simulink model "Assign_Task1and2"  (R2024a)
settings: Solver=ode1  StartTime=0.0  StopTime=simTime  FixedStep=Ts  MaxStep=Ts  RelTol=1e-3
model workspace (MAT data in the model file):
  wsw = 2000
values from neighbouring files (symbols this model uses):
  fg = 50    [Parameters.m]
  S0non = 1000e6    (= 1000000000)    [Parameters.m]
  simTime = 60    [Parameters.m]
  Ts = 20e-6    (= 2e-05)    [Parameters.m]
  Vhv = 22e3    (= 22000)    [Parameters.m]
  Vmv = 22e3    (= 22000)    [Parameters.m]
libraries: simulink_extras x8, spsCurrentMeasurementLib x6, spsGroundLib x6, spsVoltageMeasurementLib x6, spsThreePhaseParallelRLCLoadLib x5, spsPower3phInstantaneousLib x2, spsSynchronousMachinepuStandardLib x2, spsThreePhaseBreakerLib x1, spsThreePhaseSourceLib x1, sps_lib x1
settings Model: Creator=Vinicius  LastModifiedBy=citcea
settings SolverCC: AlgebraicLoopSolver=TrustRegion
settings DataIOCC: InitialState=out_EMTsteady50VSC.xFinal  SaveOperatingPoint=on  SaveOutput=off  SignalLogging=off  DSMLogging=off  TimeSaveName=t
settings OptimizationCC: BlockReduction=off
settings ModelReferenceCC: EnableRefExpFcnMdlSchedulingChecks=on
settings RTWCC: BuildConfiguration=Faster Runs  GPUComputeCapability=3.5  DLArmComputeVersion=19.05

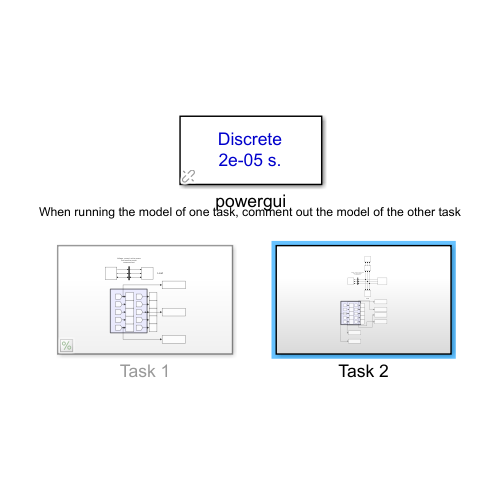
[thumbnail: Simulink's stored preview of the top-level diagram]
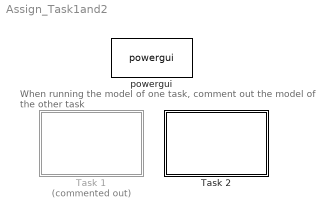
== system Assign_Task1and2 ==
  note: When running the model of one task, comment out the model of the other task
  Task 1 : Subsystem  Commented=on
  Task 2 : Subsystem
  powergui : sps_lib/powergui  Priority=1  SimulationMode=Discrete  SampleTime=Ts  frequency=60  Iterations=50  frequencyindice=50  Pbase=100e6  ErrMax=0.0001  UnitsV=kV  UnitsW=MW  buscounter=0  FunctionMessages=off  echomessages=off  EnableUseOfTLC=off  CurrentSourceSwitches=off  DisableSnubberDevices=off  DisableRonSwitches=off  DisableVfSwitches=off  DisplayEquations=off  AutomaticDiscreteSolvers=off  SolverType=Tustin/Backward Euler (TBE)  Interpol=off  ExternalGateDelay=off  methode=off  Ts=100  x0status=blocks  SPID=on  SwTol=0  HookPort=off  NonlinearTolerance=1e-4  nMaxIteration=100  ContinueOnMaxIteration=off  RestoreLinks=warning  ResistiveCurrentMeasurement=off  Frange=[0:2:500]  Ylog=off  Xlog=on  ShowGrid=off  save=off  variable=ZData  structure=0  ZoomFFT=off  StartTime=0.0  cycles=1  DisplayStyle=1  fundamental=60  FreqAxis=off  MaxFrequency=1000  frequencyindicesteady=1  RmsSteady=1  display=off

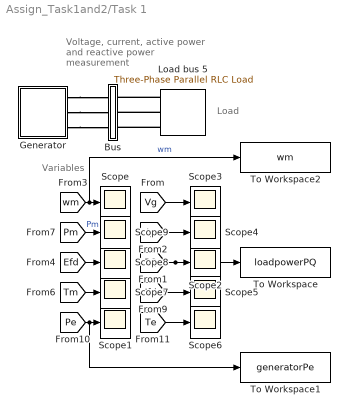
== system Assign_Task1and2/Task 1 ==
  note: Variables
  note: Voltage, current, active power and reactive power measurement
  note: Load
  Bus : Subsystem
  Generator : Subsystem
      mask Display: disp('SG')
  Load bus 5 : spsThreePhaseParallelRLCLoadLib/Three-Phase Parallel RLC Load  LConnTagsString=A|B|C  Configuration=Y (grounded)  NominalVoltage=Vmv  Vabc=[1e3 1e3 1e3]  Vabcp=[1e3 1e3 1e3]  NominalFrequency=fg  UnbalancedPower=off  ActivePower=load_active_power  InductivePower=load_inductive_power  CapacitivePower=load_capacitive_power  Pabc=[10e3 9e3 11e3]  QLabc=[100 90 110]  QCabc=[100 90 110]  Pabcp=[10e3 9e3 11e3]  QLabcp=[100 90 110]  QCabcp=[100 90 110]  Measurements=None  LoadType=constant PQ
  Scope{,1..9} (10 alike) : Scope
  To Workspace : ToWorkspace  VariableName=loadpowerPQ  SaveFormat=Timeseries  SampleTime=-1
  To Workspace1 : ToWorkspace  VariableName=generatorPe  SaveFormat=Timeseries  SampleTime=-1
  To Workspace2 : ToWorkspace  VariableName=wm  SaveFormat=Timeseries  SampleTime=-1
  wires:
  [wm] -> To Workspace2/1, Scope/1  "wm"
  [Pe] -> To Workspace1/1, Scope1/1
  [PQ] -> To Workspace/1, Scope2/1
  [Vg] -> Scope3/1
  [Ig] -> Scope4/1
  [Ifd] -> Scope5/1
  [Te] -> Scope6/1
  [Tm] -> Scope7/1
  [Efd] -> Scope8/1
  [Pm] -> Scope9/1  "Pm"
  connections:
  Load bus 5/LConn1 -- Bus/RConn1
  Load bus 5/LConn2 -- Bus/RConn2
  Generator/RConn1 -- Bus/LConn1
  Load bus 5/LConn3 -- Bus/RConn3
  Generator/RConn2 -- Bus/LConn2
  Generator/RConn3 -- Bus/LConn3

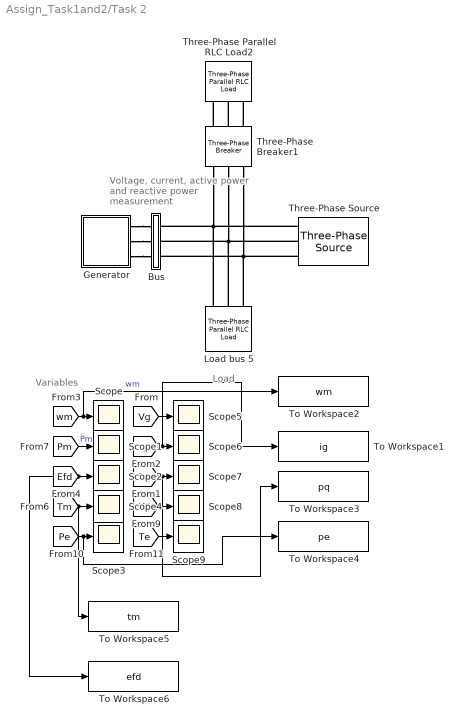
== system Assign_Task1and2/Task 2 ==
  note: Variables
  note: Voltage, current, active power and reactive power measurement
  note: Load
  Bus : Subsystem
  Generator : Subsystem
      mask Display: disp('SG')
  Load bus 5 : spsThreePhaseParallelRLCLoadLib/Three-Phase Parallel RLC Load  LConnTagsString=A|B|C  Configuration=Y (grounded)  NominalVoltage=Vmv  Vabc=[1e3 1e3 1e3]  Vabcp=[1e3 1e3 1e3]  NominalFrequency=fg  UnbalancedPower=off  ActivePower=first_load_active_power  InductivePower=first_load_inductive_power  CapacitivePower=first_load_capacitive_power  Pabc=[10e3 9e3 11e3]  QLabc=[100 90 110]  QCabc=[100 90 110]  Pabcp=[10e3 9e3 11e3]  QLabcp=[100 90 110]  QCabcp=[100 90 110]  Measurements=None  LoadType=constant PQ
  Scope{,1..9} (10 alike) : Scope
  Three-Phase Parallel RLC Load2 : spsThreePhaseParallelRLCLoadLib/Three-Phase Parallel RLC Load  LConnTagsString=A|B|C  Configuration=Y (grounded)  NominalVoltage=Vmv  Vabc=[1 1 1]*Vhv  Vabcp=[1e3 1e3 1e3]  NominalFrequency=fg  UnbalancedPower=off  ActivePower=external_load_active_power  InductivePower=external_load_inductive_power  CapacitivePower=external_load_capacitive_power  Pabc=[10 10 10]*1e6  QLabc=[1 1 1]*1e6  QCabc=[0 0 0]  Pabcp=[10e3 9e3 11e3]  QLabcp=[100 90 110]  QCabcp=[100 90 110]  Measurements=None  LoadType=constant Z
  Three-Phase Breaker1 : spsThreePhaseBreakerLib/Three-Phase Breaker  InitialState=open  SwitchA=on  SwitchB=on  SwitchC=on  SwitchTimes=simTime/2  External=off  BreakerResistance=0.001  SnubberResistance=1e7  SnubberCapacitance=inf  Measurements=None
  Three-Phase Source : spsThreePhaseSourceLib/Three-Phase Source  InternalConnection=Yg  VoltagePhases=off  Voltage=Vmv  PhaseAngle=0  Voltage_phases=[25e3 25e3 25e3]/sqrt(3)  PhaseAngles_phases=[0 -120 +120]  Frequency=50  NonIdealSource=on  SpecifyImpedance=on  Resistance=0.8929  Inductance=16.58e-3  ShortCircuitLevel=Shortcircuit_power  BaseVoltage=Vmv  XRratio=10  BusType=swing  Pref=10e3  Qref=0  Prefabc=[10e3, 10e3, 10e3]  Qrefabc=[0, 0, 0]  Qmin=-inf  Qmax=inf
  To Workspace1 : ToWorkspace  VariableName=ig  SaveFormat=Timeseries  SampleTime=-1
  To Workspace2 : ToWorkspace  VariableName=wm  SaveFormat=Timeseries  SampleTime=-1
  To Workspace3 : ToWorkspace  VariableName=pq  SaveFormat=Timeseries  SampleTime=-1
  To Workspace4 : ToWorkspace  VariableName=pe  SaveFormat=Timeseries  SampleTime=-1
  To Workspace5 : ToWorkspace  VariableName=tm  SaveFormat=Timeseries  SampleTime=-1
  To Workspace6 : ToWorkspace  VariableName=efd  SaveFormat=Timeseries  SampleTime=-1
  wires:
  [wm] -> To Workspace2/1, Scope/1  "wm"
  [Pm] -> Scope1/1  "Pm"
  [Efd] -> To Workspace6/1, Scope2/1
  [Tm] -> To Workspace5/1, Scope4/1
  [Pe] -> To Workspace4/1, Scope3/1
  [Vg] -> Scope5/1
  [Ig] -> To Workspace1/1, Scope6/1
  [PQ] -> To Workspace3/1, Scope7/1
  [Ifd] -> Scope8/1
  [Te] -> Scope9/1
  connections:
  Load bus 5/LConn1 -- Three-Phase Source/RConn1 -- Three-Phase Breaker1/LConn1 -- Bus/RConn1
  Load bus 5/LConn2 -- Three-Phase Source/RConn2 -- Three-Phase Breaker1/LConn2 -- Bus/RConn2
  Generator/RConn1 -- Bus/LConn1
  Load bus 5/LConn3 -- Three-Phase Source/RConn3 -- Three-Phase Breaker1/LConn3 -- Bus/RConn3
  Generator/RConn2 -- Bus/LConn2
  Generator/RConn3 -- Bus/LConn3
  Three-Phase Breaker1/RConn1 -- Three-Phase Parallel RLC Load2/LConn1
  Three-Phase Breaker1/RConn2 -- Three-Phase Parallel RLC Load2/LConn2
  Three-Phase Breaker1/RConn3 -- Three-Phase Parallel RLC Load2/LConn3

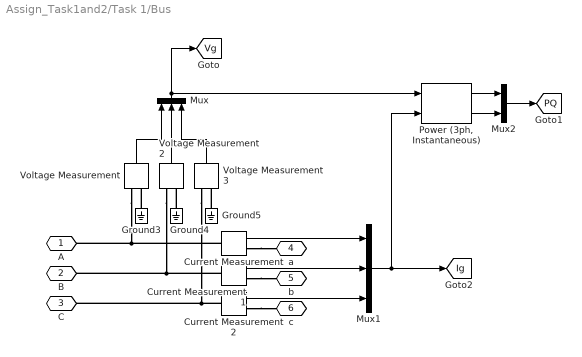
== system Assign_Task1and2/Task 1/Bus ==
  Current Measurement : spsCurrentMeasurementLib/Current Measurement  PhasorSimulation=off  OutputType=Complex  PSBequivalent=0
  Current Measurement1 : spsCurrentMeasurementLib/Current Measurement  PhasorSimulation=off  OutputType=Complex  PSBequivalent=0
  Current Measurement2 : spsCurrentMeasurementLib/Current Measurement  PhasorSimulation=off  OutputType=Complex  PSBequivalent=0
  Ground3 : spsGroundLib/Ground  LConnTagsString=a
  Ground4 : spsGroundLib/Ground  LConnTagsString=a
  Ground5 : spsGroundLib/Ground  LConnTagsString=a
  Mux : Mux  Inputs=3
  Mux1 : Mux  Inputs=3
  Mux2 : Mux  Inputs=2
  "Power (3ph, Instantaneous)" : spsPower3phInstantaneousLib/Power (3ph, Instantaneous)
  Voltage Measurement : spsVoltageMeasurementLib/Voltage Measurement  PhasorSimulation=off  OutputType=Complex  PSBequivalent=0
  Voltage Measurement2 : spsVoltageMeasurementLib/Voltage Measurement  PhasorSimulation=off  OutputType=Complex  PSBequivalent=0
  Voltage Measurement3 : spsVoltageMeasurementLib/Voltage Measurement  PhasorSimulation=off  OutputType=Complex  PSBequivalent=0
  A : PMIOPort  Side=Left
  B : PMIOPort  Port=2  Side=Left
  C : PMIOPort  Port=3  Side=Left
  a : PMIOPort  Port=4  Side=Right
  b : PMIOPort  Port=5  Side=Right
  c : PMIOPort  Port=6  Side=Right
  tag scope: Ig=global, PQ=global, Vg=global
  wires:
  Voltage Measurement3/1 -> Mux/3
  Voltage Measurement2/1 -> Mux/2
  Voltage Measurement/1 -> Mux/1
  Mux/1 -> [Vg], "Power (3ph, Instantaneous)"/1
  Current Measurement/1 -> Mux1/1
  Current Measurement1/1 -> Mux1/2
  Current Measurement2/1 -> Mux1/3
  Mux1/1 -> [Ig], "Power (3ph, Instantaneous)"/2
  "Power (3ph, Instantaneous)"/1 -> Mux2/1
  "Power (3ph, Instantaneous)"/2 -> Mux2/2
  Mux2/1 -> [PQ]
  connections:
  Ground5/LConn1 -- Voltage Measurement3/LConn2
  Current Measurement/RConn1 -- a/RConn1
  Voltage Measurement2/LConn1 -- Current Measurement1/LConn1 -- B/RConn1
  Voltage Measurement3/LConn1 -- Current Measurement2/LConn1 -- C/RConn1
  Voltage Measurement/LConn1 -- Current Measurement/LConn1 -- A/RConn1
  Ground3/LConn1 -- Voltage Measurement/LConn2
  Ground4/LConn1 -- Voltage Measurement2/LConn2
  Current Measurement1/RConn1 -- b/RConn1
  Current Measurement2/RConn1 -- c/RConn1

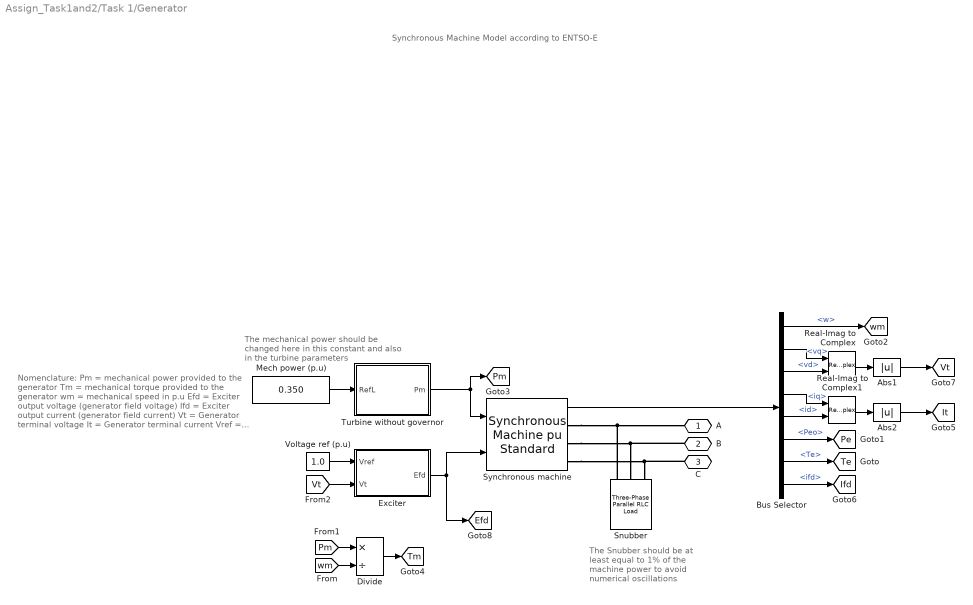
== system Assign_Task1and2/Task 1/Generator ==
  note: The Snubber should be at least equal to 1% of the machine power to avoid numerical oscillations
  note: Nomenclature:
      |
      | Pm = mechanical power provided to the generator
      | Tm = mechanical torque provided to the generator
      | wm = mechanical speed in p.u
      | Efd = Exciter output voltage (generator field voltage)
      | Ifd = Exciter output current (generator field current)
      | Vt = Generator terminal voltage
      | It = Generator terminal current
      | Vref = Voltage regulator reference signal
  note: Synchronous Machine Model according to ENTSO-E
  note: The mechanical power should be changed here in this constant and also in the turbine parameters
  Abs1 : Abs  SaturateOnIntegerOverflow=off
  Abs2 : Abs  SaturateOnIntegerOverflow=off
  Bus Selector : BusSelector  OutputSignals=w,vq,vd,iq,id,Peo,Te,ifd
  Divide : Product  Inputs=*/
  Exciter : Subsystem  mask{K=200, Ta=3, Tb=10, Te=0.05, Emin=-4, Emax=4, Vf0=1.30534}
      mask prompts: K "Controller gain (K)"; Ta "Filter derivative time constant (Ta)(sec)"; Tb "Filter delay time (Tb)(sec)"; Te "Exciter time constant (Te)(sec)"; Emin "Controller minimum output (Emin)"; Emax "Controller maximum output (Emax)"; Vf0 "Initial output (p.u)"
      mask Display:
      | disp('AVR')
      | 
      | port_label('input',1,'Vref')
      | port_label('input',2,'Vc')
      | 
      | port_label('output',1,'Efd')
  Mech power (p.u) : Constant  Value=0.350  VectorParams1D=off
  Real-Imag to Complex : RealImagToComplex
  Real-Imag to Complex1 : RealImagToComplex
  Snubber : spsThreePhaseParallelRLCLoadLib/Three-Phase Parallel RLC Load  LConnTagsString=A|B|C  Configuration=Y (grounded)  NominalVoltage=Vmv  Vabc=[1 1 1]*Vmv  Vabcp=[1e3 1e3 1e3]  NominalFrequency=fg  UnbalancedPower=off  ActivePower=0.05*S0non  InductivePower=0  CapacitivePower=0  Pabc=[10e3 10e3 10e3]  QLabc=[0 0 0]  QCabc=[0 0 0]  Pabcp=[10e3 9e3 11e3]  QLabcp=[100 90 110]  QCabcp=[100 90 110]  Measurements=None  LoadType=constant Z
  Synchronous machine : spsSynchronousMachinepuStandardLib/Synchronous Machine pu Standard  PresetModel=No  MechanicalLoad=Mechanical power Pm  ShowDetailedParameters=on  RotorType=Salient-pole  Units=per unit standard parameters  MeasurementBus=on  NominalParameters=[S0non Vmv fg]  Reactances1=[ 1.81, 0.3, 0.23, 1.76, 0.65, 0.25, 0.15 ]  Reactances2=[2.0 0.35 0.25 1.8 0.3 0.15]  dAxisTimeConstants=Short-circuit  qAxisTimeConstants=Short-circuit  TimeConstants1="[ 4.4849  0.0681  0.1  ]"  TimeConstants2=[ 8.0, 0.03, 1.0, 0.07 ]  TimeConstants3="[  4.49  0.0681  0.0513  ]"  TimeConstants4=[ 8.0, 0.03, 0.3371, 0.0295 ]  TimeConstants5=[ 1.01, 0.053, 0.1 ]  TimeConstants6=[ 1.3201, 0.023, 1.0, 0.07 ]  TimeConstants7=[0.9 0.03 0.05]  TimeConstants8=[ 1.3201, 0.0231, 0.3371, 0.0295 ]  StatorResistance=0.01  Mechanical=[6 0 2]  PolePairs=20  InitialConditions=[0 -60.0721 0.353553 0.353553 0.353553 -8.1301 -128.13 111.87 1.30534]  SetSaturation=off  Saturation=[0.6404,0.7127,0.8441,0.9214,0.9956,1.082,1.19,1.316,1.457;0.7,0.7698,0.8872,0.9466,0.9969,1.046,1.1,1.151,1.201]  LoadFlowParameters=[2 47500000 0 0 0]  TsPowergui=0  TsBlock=-1  IterativeModel=Trapezoidal non iterative  IterativeDiscreteModel=Trapezoidal non iterative  BusType=swing  Pref=475e6  Qref=0  Qmin=-inf  Qmax=inf  PLF=0  QLF=0
  Turbine without governor : Subsystem  mask{R=0.05, T1=0.5, T2=3, T3=10, Dt=0, Vmin=0, Vmax=10, P0=0.350}
      mask prompts: R "Controller droop (R)"; T1 "Governor time constant (T1)(sec)"; T2 "Turbine derivative time constant (T2)(sec)"; T3 "Turbine delay time constant (T3)(sec)"; Dt "Frictional losses factor (Dt)"; Vmin "Minimum gate limit (Vmin)(p.u)"; Vmax "Maximum gate limit (Vmax)(p.u)"; P0 "Initial power (p.u)"
      mask Display:
      | disp('Turbine')
      | 
      | port_label('input',1,'Pref')
      | 
      | port_label('output',1,'Pm')
  Voltage ref (p.u) : Constant  Value=1.0
  A : PMIOPort  Side=Right
  B : PMIOPort  Port=2  Side=Right
  C : PMIOPort  Port=3  Side=Right
  tag scope: Efd=global, Ifd=global, It=global, Pe=global, Pm=global, Te=global, Tm=global, Vt=global, wm=global
  wires:
  Exciter/1(Efd) -> Synchronous machine/2, [Efd]
  Voltage ref (p.u)/1 -> Exciter/1(Vref)
  Turbine without governor/1(Pm) -> Synchronous machine/1, [Pm]
  Mech power (p.u)/1 -> Turbine without governor/1(RefL)
  [Pm] -> Divide/1
  [wm] -> Divide/2
  Divide/1 -> [Tm]
  Bus Selector/3 -> Real-Imag to Complex/2  "<vd>"
  Abs2/1 -> [It]
  Real-Imag to Complex1/1 -> Abs2/1
  Real-Imag to Complex/1 -> Abs1/1
  Bus Selector/5 -> Real-Imag to Complex1/2  "<id>"
  Bus Selector/1 -> [wm]  "<w>"
  Bus Selector/7 -> [Te]  "<Te>"
  Bus Selector/2 -> Real-Imag to Complex/1  "<vq>"
  Bus Selector/6 -> [Pe]  "<Peo>"
  Bus Selector/4 -> Real-Imag to Complex1/1  "<iq>"
  Synchronous machine/1 -> Bus Selector/1
  Bus Selector/8 -> [Ifd]  "<ifd>"
  Abs1/1 -> [Vt]
  [Vt] -> Exciter/2(Vt)
  connections:
  B/RConn1 -- Synchronous machine/RConn2 -- Snubber/LConn2
  C/RConn1 -- Synchronous machine/RConn3 -- Snubber/LConn3
  Snubber/LConn1 -- Synchronous machine/RConn1 -- A/RConn1

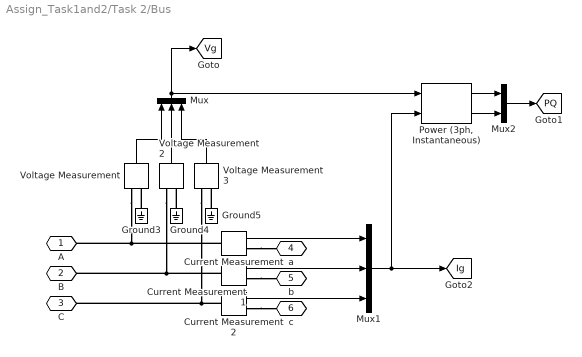
== system Assign_Task1and2/Task 2/Bus ==
  Current Measurement : spsCurrentMeasurementLib/Current Measurement  PhasorSimulation=off  OutputType=Complex  PSBequivalent=0
  Current Measurement1 : spsCurrentMeasurementLib/Current Measurement  PhasorSimulation=off  OutputType=Complex  PSBequivalent=0
  Current Measurement2 : spsCurrentMeasurementLib/Current Measurement  PhasorSimulation=off  OutputType=Complex  PSBequivalent=0
  Ground3 : spsGroundLib/Ground  LConnTagsString=a
  Ground4 : spsGroundLib/Ground  LConnTagsString=a
  Ground5 : spsGroundLib/Ground  LConnTagsString=a
  Mux : Mux  Inputs=3
  Mux1 : Mux  Inputs=3
  Mux2 : Mux  Inputs=2
  "Power (3ph, Instantaneous)" : spsPower3phInstantaneousLib/Power (3ph, Instantaneous)
  Voltage Measurement : spsVoltageMeasurementLib/Voltage Measurement  PhasorSimulation=off  OutputType=Complex  PSBequivalent=0
  Voltage Measurement2 : spsVoltageMeasurementLib/Voltage Measurement  PhasorSimulation=off  OutputType=Complex  PSBequivalent=0
  Voltage Measurement3 : spsVoltageMeasurementLib/Voltage Measurement  PhasorSimulation=off  OutputType=Complex  PSBequivalent=0
  A : PMIOPort  Side=Left
  B : PMIOPort  Port=2  Side=Left
  C : PMIOPort  Port=3  Side=Left
  a : PMIOPort  Port=4  Side=Right
  b : PMIOPort  Port=5  Side=Right
  c : PMIOPort  Port=6  Side=Right
  tag scope: Ig=global, PQ=global, Vg=global
  wires:
  Voltage Measurement3/1 -> Mux/3
  Voltage Measurement2/1 -> Mux/2
  Voltage Measurement/1 -> Mux/1
  Mux/1 -> [Vg], "Power (3ph, Instantaneous)"/1
  Current Measurement/1 -> Mux1/1
  Current Measurement1/1 -> Mux1/2
  Current Measurement2/1 -> Mux1/3
  Mux1/1 -> [Ig], "Power (3ph, Instantaneous)"/2
  "Power (3ph, Instantaneous)"/1 -> Mux2/1
  "Power (3ph, Instantaneous)"/2 -> Mux2/2
  Mux2/1 -> [PQ]
  connections:
  Ground5/LConn1 -- Voltage Measurement3/LConn2
  Current Measurement/RConn1 -- a/RConn1
  Voltage Measurement2/LConn1 -- Current Measurement1/LConn1 -- B/RConn1
  Voltage Measurement3/LConn1 -- Current Measurement2/LConn1 -- C/RConn1
  Voltage Measurement/LConn1 -- Current Measurement/LConn1 -- A/RConn1
  Ground3/LConn1 -- Voltage Measurement/LConn2
  Ground4/LConn1 -- Voltage Measurement2/LConn2
  Current Measurement1/RConn1 -- b/RConn1
  Current Measurement2/RConn1 -- c/RConn1

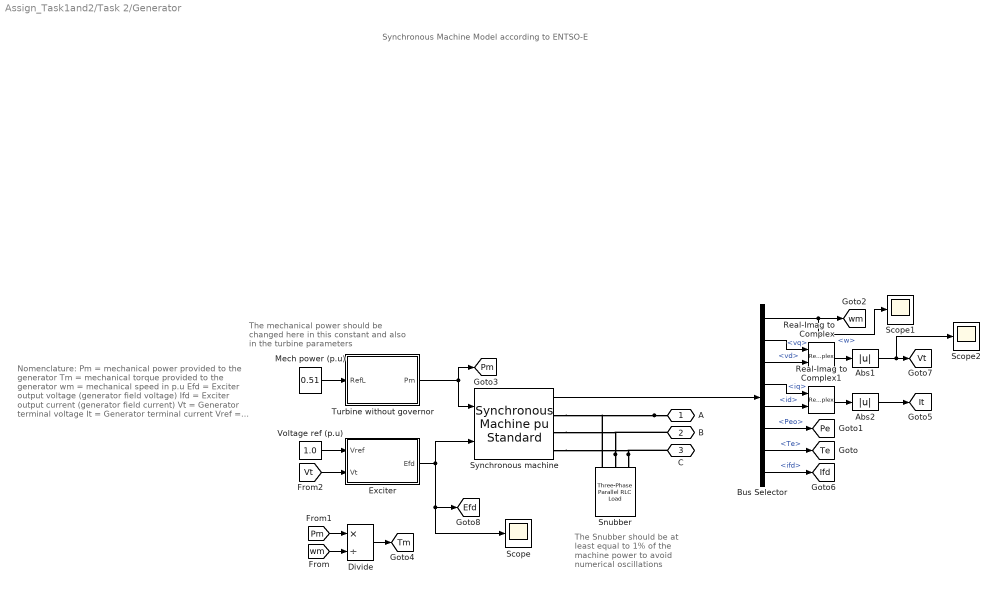
== system Assign_Task1and2/Task 2/Generator ==
  note: The Snubber should be at least equal to 1% of the machine power to avoid numerical oscillations
  note: Nomenclature:
      |
      | Pm = mechanical power provided to the generator
      | Tm = mechanical torque provided to the generator
      | wm = mechanical speed in p.u
      | Efd = Exciter output voltage (generator field voltage)
      | Ifd = Exciter output current (generator field current)
      | Vt = Generator terminal voltage
      | It = Generator terminal current
      | Vref = Voltage regulator reference signal
  note: Synchronous Machine Model according to ENTSO-E
  note: The mechanical power should be changed here in this constant and also in the turbine parameters
  Abs1 : Abs  SaturateOnIntegerOverflow=off
  Abs2 : Abs  SaturateOnIntegerOverflow=off
  Bus Selector : BusSelector  OutputSignals=w,vq,vd,iq,id,Peo,Te,ifd
  Divide : Product  Inputs=*/
  Exciter : Subsystem  mask{K=200, Ta=3, Tb=10, Te=0.05, Emin=-4, Emax=4, Vf0=1.6}
      mask prompts: K "Controller gain (K)"; Ta "Filter derivative time constant (Ta)(sec)"; Tb "Filter delay time (Tb)(sec)"; Te "Exciter time constant (Te)(sec)"; Emin "Controller minimum output (Emin)"; Emax "Controller maximum output (Emax)"; Vf0 "Initial output (p.u)"
      mask Display:
      | disp('AVR')
      | 
      | port_label('input',1,'Vref')
      | port_label('input',2,'Vc')
      | 
      | port_label('output',1,'Efd')
  Mech power (p.u) : Constant  Value=0.51  VectorParams1D=off
  Real-Imag to Complex : RealImagToComplex
  Real-Imag to Complex1 : RealImagToComplex
  Scope : Scope
  Scope1 : Scope
  Scope2 : Scope
  Snubber : spsThreePhaseParallelRLCLoadLib/Three-Phase Parallel RLC Load  LConnTagsString=A|B|C  Configuration=Y (grounded)  NominalVoltage=Vmv  Vabc=[1 1 1]*Vmv  Vabcp=[1e3 1e3 1e3]  NominalFrequency=fg  UnbalancedPower=off  ActivePower=0.01*S0non  InductivePower=0  CapacitivePower=0  Pabc=[10e3 10e3 10e3]  QLabc=[0 0 0]  QCabc=[0 0 0]  Pabcp=[10e3 9e3 11e3]  QLabcp=[100 90 110]  QCabcp=[100 90 110]  Measurements=None  LoadType=constant Z
  Synchronous machine : spsSynchronousMachinepuStandardLib/Synchronous Machine pu Standard  PresetModel=No  MechanicalLoad=Mechanical power Pm  ShowDetailedParameters=on  RotorType=Salient-pole  Units=per unit standard parameters  MeasurementBus=on  NominalParameters=[S0non Vmv fg]  Reactances1=[ 1.81, 0.3, 0.23, 1.76, 0.65, 0.25, 0.15 ]  Reactances2=[2.0 0.35 0.25 1.8 0.3 0.15]  dAxisTimeConstants=Short-circuit  qAxisTimeConstants=Short-circuit  TimeConstants1="[ 4.4849  0.0681  0.1  ]"  TimeConstants2=[ 8.0, 0.03, 1.0, 0.07 ]  TimeConstants3="[  4.49  0.0681  0.0513  ]"  TimeConstants4=[ 8.0, 0.03, 0.3371, 0.0295 ]  TimeConstants5=[ 1.01, 0.053, 0.1 ]  TimeConstants6=[ 1.3201, 0.023, 1.0, 0.07 ]  TimeConstants7=[0.9 0.03 0.05]  TimeConstants8=[ 1.3201, 0.0231, 0.3371, 0.0295 ]  StatorResistance=0.01  Mechanical=[6 0 2]  PolePairs=20  InitialConditions=[0 -60.0721 0.353553 0.353553 0.353553 -8.1301 -128.13 111.87 1.6]  SetSaturation=off  Saturation=[0.6404,0.7127,0.8441,0.9214,0.9956,1.082,1.19,1.316,1.457;0.7,0.7698,0.8872,0.9466,0.9969,1.046,1.1,1.151,1.201]  LoadFlowParameters=[2 47500000 0 0 0]  TsPowergui=0  TsBlock=-1  IterativeModel=Trapezoidal non iterative  IterativeDiscreteModel=Trapezoidal non iterative  BusType=swing  Pref=475e6  Qref=0  Qmin=-inf  Qmax=inf  PLF=0  QLF=0
  Turbine without governor : Subsystem  mask{R=0.05, T1=0.5, T2=3, T3=10, Dt=0, Vmin=0, Vmax=10, P0=0.51}
      mask prompts: R "Controller droop (R)"; T1 "Governor time constant (T1)(sec)"; T2 "Turbine derivative time constant (T2)(sec)"; T3 "Turbine delay time constant (T3)(sec)"; Dt "Frictional losses factor (Dt)"; Vmin "Minimum gate limit (Vmin)(p.u)"; Vmax "Maximum gate limit (Vmax)(p.u)"; P0 "Initial power (p.u)"
      mask Display:
      | disp('Turbine')
      | 
      | port_label('input',1,'Pref')
      | 
      | port_label('output',1,'Pm')
  Voltage ref (p.u) : Constant  Value=1.0
  A : PMIOPort  Side=Right
  B : PMIOPort  Port=2  Side=Right
  C : PMIOPort  Port=3  Side=Right
  tag scope: Efd=global, Ifd=global, It=global, Pe=global, Pm=global, Te=global, Tm=global, Vt=global, wm=global
  wires:
  Exciter/1(Efd) -> Synchronous machine/2, Scope/1, [Efd]
  Voltage ref (p.u)/1 -> Exciter/1(Vref)
  Turbine without governor/1(Pm) -> Synchronous machine/1, [Pm]
  Mech power (p.u)/1 -> Turbine without governor/1(RefL)
  [Pm] -> Divide/1
  [wm] -> Divide/2
  Divide/1 -> [Tm]
  Bus Selector/3 -> Real-Imag to Complex/2  "<vd>"
  Abs2/1 -> [It]
  Real-Imag to Complex1/1 -> Abs2/1
  Real-Imag to Complex/1 -> Abs1/1
  Bus Selector/5 -> Real-Imag to Complex1/2  "<id>"
  Bus Selector/1 -> Scope1/1, [wm]  "<w>"
  Bus Selector/7 -> [Te]  "<Te>"
  Bus Selector/2 -> Real-Imag to Complex/1  "<vq>"
  Bus Selector/6 -> [Pe]  "<Peo>"
  Bus Selector/4 -> Real-Imag to Complex1/1  "<iq>"
  Synchronous machine/1 -> Bus Selector/1
  Bus Selector/8 -> [Ifd]  "<ifd>"
  Abs1/1 -> Scope2/1, [Vt]
  [Vt] -> Exciter/2(Vt)
  connections:
  Snubber/LConn2 -- B/RConn1 -- Synchronous machine/RConn2
  Snubber/LConn3 -- C/RConn1 -- Synchronous machine/RConn3
  A/RConn1 -- Snubber/LConn1 -- Synchronous machine/RConn1

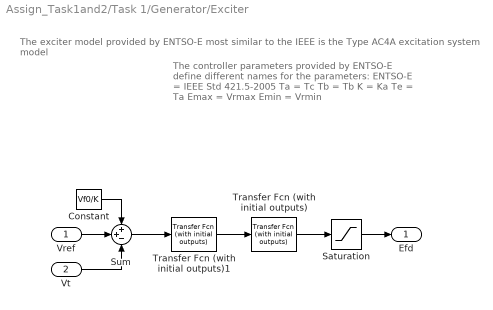
== system Assign_Task1and2/Task 1/Generator/Exciter ==
  note: The controller parameters provided by ENTSO-E
      | define different names for the parameters:
      |
      | ENTSO-E = IEEE Std 421.5-2005
      | Ta = Tc
      | Tb = Tb
      | K = Ka
      | Te = Ta
      | Emax = Vrmax
      | Emin = Vrmin
  note: The exciter model provided by ENTSO-E most similar to the IEEE is the Type AC4A excitation system model
  Vref : Inport
  Vt : Inport  Port=2
  Constant : Constant  Value=Vf0/K
  Saturation : Saturate  UpperLimit=Emax  LowerLimit=Emin
  Sum : Sum  Inputs=++-
  Transfer Fcn (with initial outputs) : simulink_extras/Additional Linear/Transfer Fcn (with initial outputs)  N=[K]  D=[Te 1]  Y0=Vf0  U0=Vf0/K
  Transfer Fcn (with initial outputs)1 : simulink_extras/Additional Linear/Transfer Fcn (with initial outputs)  N=[Ta 1]  D=[Tb 1]  Y0=Vf0/K  U0=Vf0/K
  Efd : Outport
  wires:
  Saturation/1 -> Efd/1
  Transfer Fcn (with initial outputs)1/1 -> Transfer Fcn (with initial outputs)/1
  Sum/1 -> Transfer Fcn (with initial outputs)1/1
  Transfer Fcn (with initial outputs)/1 -> Saturation/1
  Vt/1 -> Sum/3
  Vref/1 -> Sum/2
  Constant/1 -> Sum/1

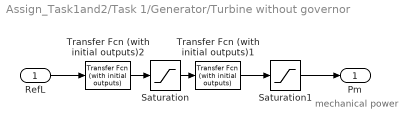
== system Assign_Task1and2/Task 1/Generator/Turbine without governor ==
  note: mechanical power
  RefL : Inport
  Saturation : Saturate  UpperLimit=Vmax  LowerLimit=Vmin
  Saturation1 : Saturate  UpperLimit=1
  Transfer Fcn (with initial outputs)1 : simulink_extras/Additional Linear/Transfer Fcn (with initial outputs)  N=[T2 1]  D=[T3 1]  Y0=P0  U0=P0
  Transfer Fcn (with initial outputs)2 : simulink_extras/Additional Linear/Transfer Fcn (with initial outputs)  N=[1]  D=[T1 1]  Y0=P0  U0=P0
  Pm : Outport
  wires:
  Transfer Fcn (with initial outputs)1/1 -> Saturation1/1
  Saturation/1 -> Transfer Fcn (with initial outputs)1/1
  Transfer Fcn (with initial outputs)2/1 -> Saturation/1
  RefL/1 -> Transfer Fcn (with initial outputs)2/1
  Saturation1/1 -> Pm/1

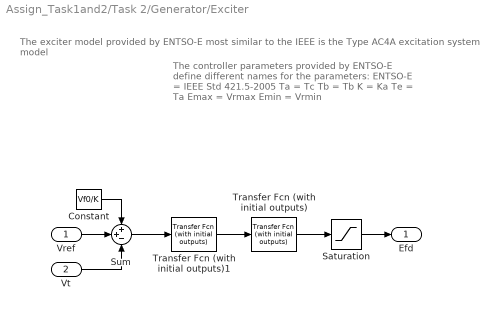
== system Assign_Task1and2/Task 2/Generator/Exciter ==
  note: The controller parameters provided by ENTSO-E
      | define different names for the parameters:
      |
      | ENTSO-E = IEEE Std 421.5-2005
      | Ta = Tc
      | Tb = Tb
      | K = Ka
      | Te = Ta
      | Emax = Vrmax
      | Emin = Vrmin
  note: The exciter model provided by ENTSO-E most similar to the IEEE is the Type AC4A excitation system model
  Vref : Inport
  Vt : Inport  Port=2
  Constant : Constant  Value=Vf0/K
  Saturation : Saturate  UpperLimit=Emax  LowerLimit=Emin
  Sum : Sum  Inputs=++-
  Transfer Fcn (with initial outputs) : simulink_extras/Additional Linear/Transfer Fcn (with initial outputs)  N=[K]  D=[Te 1]  Y0=Vf0  U0=Vf0/K
  Transfer Fcn (with initial outputs)1 : simulink_extras/Additional Linear/Transfer Fcn (with initial outputs)  N=[Ta 1]  D=[Tb 1]  Y0=Vf0/K  U0=Vf0/K
  Efd : Outport
  wires:
  Saturation/1 -> Efd/1
  Transfer Fcn (with initial outputs)1/1 -> Transfer Fcn (with initial outputs)/1
  Sum/1 -> Transfer Fcn (with initial outputs)1/1
  Transfer Fcn (with initial outputs)/1 -> Saturation/1
  Vt/1 -> Sum/3
  Vref/1 -> Sum/2
  Constant/1 -> Sum/1

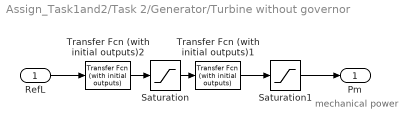
== system Assign_Task1and2/Task 2/Generator/Turbine without governor ==
  note: mechanical power
  RefL : Inport
  Saturation : Saturate  UpperLimit=Vmax  LowerLimit=Vmin
  Saturation1 : Saturate  UpperLimit=1
  Transfer Fcn (with initial outputs)1 : simulink_extras/Additional Linear/Transfer Fcn (with initial outputs)  N=[T2 1]  D=[T3 1]  Y0=P0  U0=P0
  Transfer Fcn (with initial outputs)2 : simulink_extras/Additional Linear/Transfer Fcn (with initial outputs)  N=[1]  D=[T1 1]  Y0=P0  U0=P0
  Pm : Outport
  wires:
  Transfer Fcn (with initial outputs)1/1 -> Saturation1/1
  Saturation/1 -> Transfer Fcn (with initial outputs)1/1
  Transfer Fcn (with initial outputs)2/1 -> Saturation/1
  RefL/1 -> Transfer Fcn (with initial outputs)2/1
  Saturation1/1 -> Pm/1
